simulink model "script_model_modified"  (R2023a)
settings: Solver=FixedStepAuto  StartTime=0.0  StopTime=10.0  FixedStep=ts  RelTol=1e-3
values from neighbouring files (symbols this model uses):
  Q = diag([0.1, 5, 0.1, 5])    [mpcdef.m]
  R = 1e-7    (= 1e-07)    [mpcdef.m]
  T_c = 6    [mpcdef.m]
  T_p = 12    [mpcdef.m]
  ts = 0.01    [mpcdef.m]
  u_lb = -2500    [mpcdef.m]
  u_ub = 2500    [mpcdef.m]
undefined symbols (not defined in the file or in its folder): A_d, B_d, C_d, D_d, road_disturbance_dot_padded
settings Model: Creator=Adham  LastModifiedBy=Adham

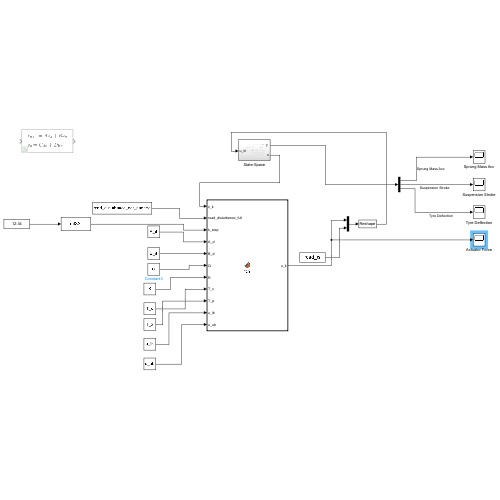
[thumbnail: Simulink's stored preview of the top-level diagram]
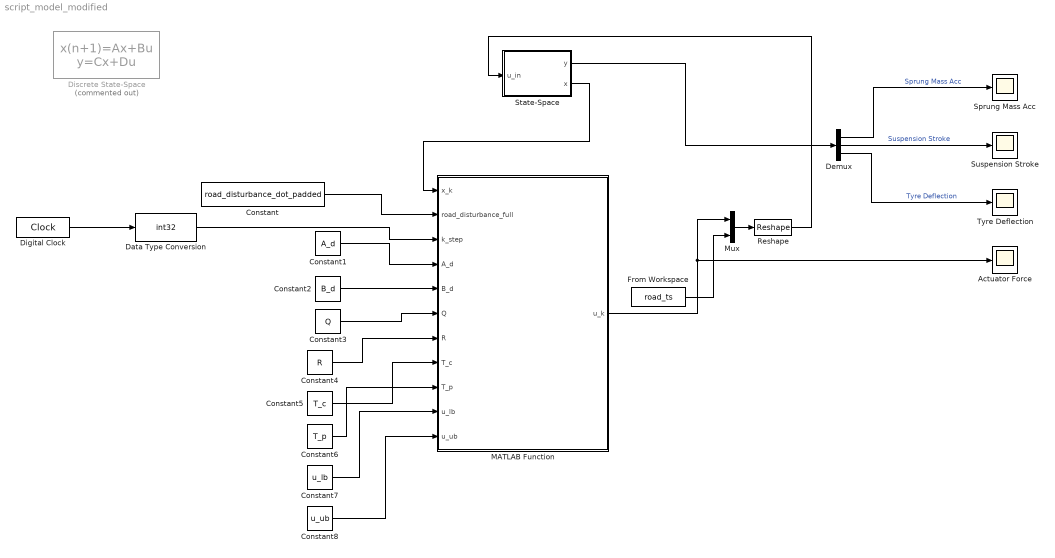
== system script_model_modified ==
  Actuator Force : Scope
  Constant : Constant  Value=road_disturbance_dot_padded
  Constant1 : Constant  Value=A_d
  Constant2 : Constant  Value=B_d
  Constant3 : Constant  Value=Q
  Constant4 : Constant  Value=R
  Constant5 : Constant  Value=T_c
  Constant6 : Constant  Value=T_p
  Constant7 : Constant  Value=u_lb
  Constant8 : Constant  Value=u_ub
  Data Type Conversion : DataTypeConversion  OutDataTypeStr=int32  SaturateOnIntegerOverflow=off  RndMeth=Floor
  Demux : Demux  Outputs=3
  Digital Clock : DigitalClock  SampleTime=ts
  Discrete State-Space : DiscreteStateSpace  Commented=on  A=A_d  B=B_d  C=C_d  D=D_d  SampleTime=ts
  From Workspace : FromWorkspace  VariableName=road_ts
  MATLAB Function : MATLAB Function  TreatAsAtomicUnit=on
  Mux : Mux  Inputs=2
  Reshape : Reshape  OutputDimensionality=Customize  OutputDimensions=[2 1]
  Sprung Mass Acc : Scope
  State-Space : Subsystem
  Suspension Stroke : Scope
  Tyre Deflection : Scope
  wires:
  From Workspace/1 -> Mux/2
  State-Space/2(x) -> MATLAB Function/1(x_k)
  MATLAB Function/1(u_k) -> Mux/1, Actuator Force/1
  Mux/1 -> Reshape/1
  Reshape/1 -> State-Space/1(u_in)
  State-Space/1("y ") -> Demux/1
  Demux/1 -> Sprung Mass Acc/1  "Sprung Mass Acc"
  Demux/2 -> Suspension Stroke/1  "Suspension Stroke"
  Demux/3 -> Tyre Deflection/1  "Tyre Deflection"
  Constant/1 -> MATLAB Function/2(road_disturbance_full)
  Digital Clock/1 -> Data Type Conversion/1
  Constant8/1 -> MATLAB Function/11(u_ub)
  Constant7/1 -> MATLAB Function/10(u_lb)
  Constant6/1 -> MATLAB Function/9(T_p)
  Constant5/1 -> MATLAB Function/8(T_c)
  Constant4/1 -> MATLAB Function/7(R)
  Constant3/1 -> MATLAB Function/6(Q)
  Constant2/1 -> MATLAB Function/5(B_d)
  Constant1/1 -> MATLAB Function/4(A_d)
  Data Type Conversion/1 -> MATLAB Function/3(k_step)

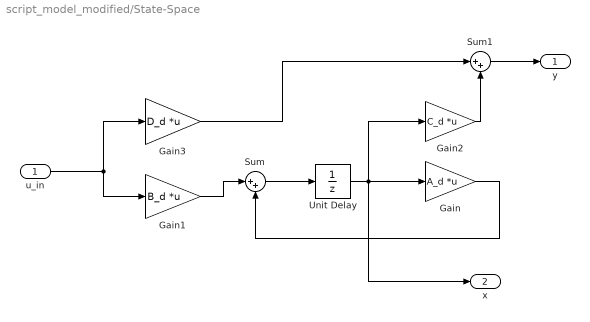
== system script_model_modified/State-Space ==
  u_in : Inport
  Gain : Gain  Gain=A_d  Multiplication=Matrix(K*u)
  Gain1 : Gain  Gain=B_d  Multiplication=Matrix(K*u)
  Gain2 : Gain  Gain=C_d  Multiplication=Matrix(K*u)
  Gain3 : Gain  Gain=D_d  Multiplication=Matrix(K*u)
  Sum : Sum  Inputs=|++
  Sum1 : Sum  Inputs=|++
  Unit Delay : UnitDelay  InitialCondition=zeros(4,1)  SampleTime=ts  HasFrameUpgradeWarning=on
  "y " : Outport
  x : Outport  Port=2
  wires:
  Gain1/1 -> Sum/1
  Sum/1 -> Unit Delay/1
  Unit Delay/1 -> x/1, Gain/1, Gain2/1
  Gain3/1 -> Sum1/1
  Gain/1 -> Sum/2
  Sum1/1 -> "y "/1
  Gain2/1 -> Sum1/2
  u_in/1 -> Gain3/1, Gain1/1

== matlab function script_model_modified/MATLAB Function ==
  data: x_k input; u_k output; road_disturbance_full input; k_step input; A_d input; B_d input; Q input; R input; T_c input; T_p input; u_lb input; u_ub input
function u_k = fcn(x_k, road_disturbance_full, k_step, A_d, B_d, Q, R, T_c, T_p, u_lb, u_ub)
% This function implements the proactive MPC logic for a single time step.

% --- Create the Road Preview (Simplified) ---
% Create the preview window by slicing the pre-padded array.
% We add 1 to k_step to convert Simulink's 0-based step to MATLAB's 1-based index.
start_index = k_step + 1;
end_index = k_step + T_p;
road_preview = road_disturbance_full(start_index : end_index);

% --- Optimization Problem Setup ---
u0 = zeros(T_c, 1);
lb = repmat(u_lb, T_c, 1);
ub = repmat(u_ub, T_c, 1);

cost_func = @(u) mpc_cost_function(u, A_d, B_d, Q, R, x_k, road_preview, T_c, T_p);
options = optimoptions('fmincon','Display','none','Algorithm','sqp');
u_optimal = fmincon(cost_func, u0, [], [], [], [], lb, ub, [], options);

u_k = u_optimal(1);

end

function cost = mpc_cost_function(u_seq, A_d, B_d, Q, R, x_0, z_road, T_c, T_p)
    cost = 0;
    x_k = x_0;
    
    for i = 1:T_c
        u_k = u_seq(i);
        dist_k = z_road(i);
        cost = cost + x_k'*Q*x_k + u_k'*R*u_k;
        x_k = A_d*x_k + B_d*[u_k; dist_k];
    end
    
    for i = T_c+1 : T_p
        dist_k = z_road(i);
        cost = cost + x_k'*Q*x_k;
        x_k = A_d*x_k + B_d*[0; dist_k];
    end
    cost = cost + x_k'*Q*x_k;
end
